simulink model "ims_Build5pt1g_tj"  (R2020b)
settings: Solver=FixedStepDiscrete  StartTime=0.0  StopTime=180  FixedStep=fem.Ts  RelTol=1e-4
InitFcn:
  | %
  | % Initialization callback function
  | %
  | 
  | try
  |    fprintf('\n New GMT IMS version!\n');
  | 
  |    % Get Simulink model directory
  |    [filepath,name,ext] = fileparts(which(bdroot));
  | 
  |    if ~strcmp(filepath,pwd)
  |       fprintf('\n Changing current directory to \n %s \n',filepath);
  |       cd(filepath);
  |    end
  | 
  |    %
  |    if(~exist('IMLoads','var'))
  |        warning('Simulation model assumes wind load is loaded...');
  |    end
  | catch
  |    warning('Running the InitFcn from puSimulate script');
  | end
values from neighbouring files (symbols this model uses):
  az = zeros(N,1)    [eval_trajectories.m]
  az_ff_en = 1    [load_IMS_5pt1g_tj.m]    (also in load_IMS_5pt1h_tj.m = 0)
  el = az    [eval_trajectories.m]
  el_ff_en = 1    [load_IMS_5pt1g_tj.m]    (also in load_IMS_5pt1h_tj.m = 0)
  fem =     [controls_5pt1g1K_z00_llTT_oad.mat]    (also in controls_5pt1g1K_z30_llTT_oad.mat)
  FEM_Ts = 1/1e3    (= 0.001)    [load_IMS_5pt1g_tj.m]    (also in load_IMS_5pt1h_tj.m)
  gir = az    [eval_trajectories.m]
  gir_ff_en = 1    [load_IMS_5pt1g_tj.m]    (also in load_IMS_5pt1h_tj.m = 0)
  H_tj = tf(1,[2*pi*0.1, 1])    [eval_trajectories.m]    (also in load_IMS_5pt1g_tj.m = c2d(Htjf,FEM_Ts, 'foh'); load_IMS_5pt1h_tj.m = c2d(Htjf,FEM_Ts, 'foh'))
  Hkin_fsm = Phi(fsm_out,1:3) * Phi_mnt_pinv    [compute_Hkin.m]
  Hkin_hp = Phi(hp_out,1:3) * Phi_mnt_pinv    [compute_Hkin.m]
  Hkin_m12 = [Phi(m1_out,1:3); Phi(m2_out,1:3)] * Phi_mnt_pinv    [compute_Hkin.m]    (also in eval_tjs.m = [Phi(m1_out,1:3); Phi(m2_out,1:3)] * pinv(Phi_mnt_enc))
  Hkin_m2p = Phi(m2p_out,1:3) * Phi_mnt_pinv    [compute_Hkin.m]
  Hkin_pmtnodes = Phi(pmt_out,1:3) * Phi_mnt_pinv    [compute_Hkin.m]    (also in eval_tjs.m = Phi(pmt_out,1:3) * pinv(Phi_mnt_enc))
  m1olf_en = 0    [load_IMS_5pt1g_tj.m]    (also in load_IMS_5pt1h_tj.m)
  m1sys =     [controls_5pt1g1K_z00_llTT_oad.mat]    (also in controls_5pt1g1K_z30_llTT_oad.mat)
  m2_pos_en = 0    [load_IMS_5pt1g_tj.m]    (also in load_IMS_5pt1h_tj.m)
  m2pos =     [controls_5pt1g1K_z00_llTT_oad.mat]    (also in controls_5pt1g1K_z30_llTT_oad.mat)
  m2pzt =     [controls_5pt1g1K_z00_llTT_oad.mat]    (also in controls_5pt1g1K_z30_llTT_oad.mat)
  m2PZT_en = 0    [load_IMS_5pt1g_tj.m]    (also in load_IMS_5pt1h_tj.m)
  mntFBc_en = 1    [load_IMS_5pt1g_tj.m]    (also in load_IMS_5pt1h_tj.m)
  mount =     [controls_5pt1g1K_z00_llTT_oad.mat]    (also in controls_5pt1g1K_z30_llTT_oad.mat; eval_tjs.m = mountY)
  om2 = (2*pi*eigenfrequencies).^2    [load_IMS_5pt1g_tj.m]    (also in load_IMS_5pt1h_tj.m)
  PG = zeros(length(om2),6)    [load_IMS_5pt1g_tj.m]    (also in load_IMS_5pt1h_tj.m)
  phiB = Phim(indDesInputs,:)'    [load_IMS_5pt1g_tj.m]    (also in load_IMS_5pt1h_tj.m)
  phiC = Phi(indDesOutputs,:)    [load_IMS_5pt1g_tj.m]    (also in load_IMS_5pt1h_tj.m)
  pmt1 = dlmread(pmt1_fname,',',[14,3,27,302])    [eval_tjs.m]    (also in eval_tjs_rtf_variants.m; load_IMS_5pt1g_tj.m; load_IMS_5pt1h_tj.m)
  pmt2 = dlmread(pmt2_fname,',',[14,3,10,302])    [eval_tjs.m]    (also in eval_tjs_rtf_variants.m; load_IMS_5pt1g_tj.m; load_IMS_5pt1h_tj.m)
  Psi_ss = gainMatrix(indDesOutputs,indDesInputs) - K_ss    [load_IMS_5pt1g_tj.m]    (also in load_IMS_5pt1h_tj.m)
  Psi_ssTs = 1/1000    (= 0.001)    [load_IMS_5pt1g_tj.m]    (also in load_IMS_5pt1h_tj.m)
  twice_zom = adjDamp*twice_zom    [load_IMS_5pt1g_tj.m]    (also in load_IMS_5pt1h_tj.m)
undefined symbols (not defined in the file or in its folder): DiscIntNeverNeededParam, magnitude
libraries: ims_block_library x20, simulink x1
(part 1 of 2)
settings Model: SimulationMode=accelerator  Creator=RRomano  LastModifiedBy=rromano
settings SolverCC: MaxConsecutiveMinStep=10  ZeroCrossAlgorithm=Adaptive
settings DataIOCC: SaveOutput=off  SignalLogging=off  DSMLogging=off  SaveTime=off  ReturnWorkspaceOutputs=off
settings OptimizationCC: DefaultParameterBehavior=Inlined  StrengthReduction=on  PassReuseOutputArgsAs=Individual arguments  EfficientMapNaN2IntZero=off  SimCompilerOptimization=on  AccelVerboseBuild=on  OptimizeBlockOrder=speed  OptimizationPriority=Speed  OptimizationCustomize=off  MultiThreadedLoops=on  EfficientTunableParamExpr=on
settings DebuggingCC: SignalInfNanChecking=warning  InheritedTsInSrcMsg=none  ParameterTunabilityLossMsg=error  SFUnexpectedBacktrackingDiag=warning  SFNoUnconditionalDefaultTransitionDiag=warning  SFExecutionAtInitializationDiag=none  ArithmeticOperatorsInVariantConditions=warning
settings HardwareCC: ProdBitPerLong=64  ProdHWDeviceType=Intel->x86-64 (Linux 64)  TargetBitPerLong=64  TargetBitPerPointer=64  TargetBitPerSizeT=64  TargetBitPerPtrDiffT=64  TargetLongLongMode=on  TargetIntDivRoundTo=Zero  TargetEndianess=LittleEndian  TargetWordSize=64  TargetHWDeviceType=MATLAB Host  ProdEqTarget=off
settings SFSimCC: SimUseLocalCustomCode=off  MATLABDynamicMemAlloc=off  CustomCodeUndefinedFunction=UseInterfaceOnly
settings RTWCC: Description=Embedded Coder  SystemTargetFile=ert.tlc  GenCodeOnly=on  TemplateMakefile=ert_default_tmf  GenerateReport=on  BuildConfiguration=Faster Runs  IncludeHyperlinkInReport=on  GenerateTraceInfo=on  GenerateTraceReport=on  GenerateTraceReportSl=on  GenerateTraceReportSf=on  GenerateTraceReportEml=on
settings CodeAppCC: ForceParamTrailComments=on  IgnoreCustomStorageClasses=off  MaxIdLength=128  OperatorAnnotations=on  SimulinkDataObjDesc=on  SFDataObjDesc=on  InsertBlockDesc=on  MATLABSourceComments=on
settings ERTTargetCC: GenerateSampleERTMain=on  InlinedParameterPlacement=NonHierarchical  ERTCustomFileTemplate=example_file_process.tlc
settings ConfigComp: CovMetricSettings=dw  CovSaveCumulativeToWorkspaceVar=on  CovSaveSingleToWorkspaceVar=on  CovExternalEMLEnable=off

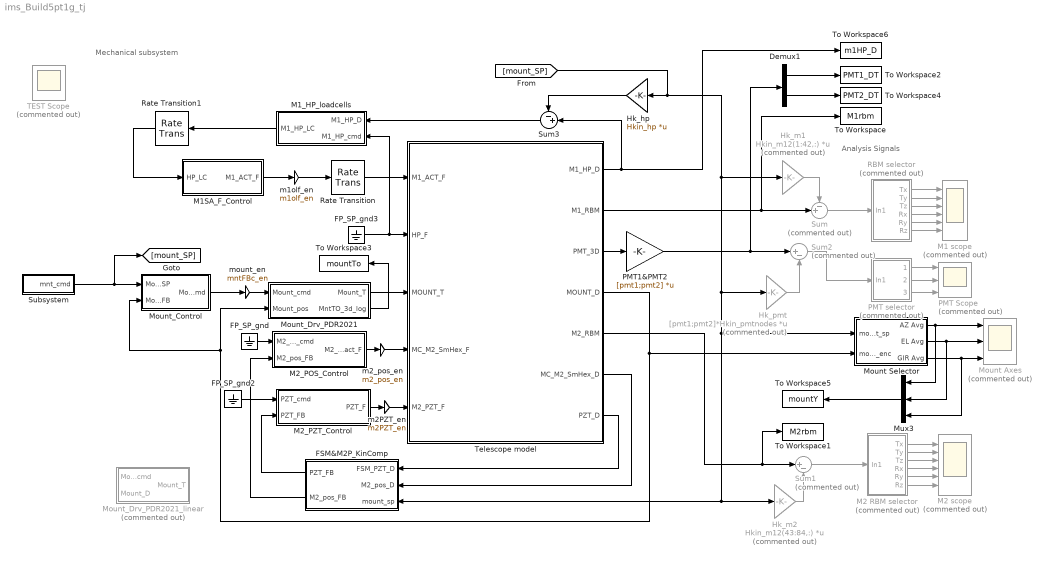
== system ims_Build5pt1g_tj ==
  note: Analysis Signals
  note: Mechanical subsystem
  Demux1 : Demux  Outputs=[14,7]
  FP_SP_gnd : Ground
  FP_SP_gnd2 : Ground
  FP_SP_gnd3 : Ground
  FSM&M2P_KinComp : Subsystem
  Hk_hp : Gain  Gain=Hkin_hp  Multiplication=Matrix(K*u)
  Hk_m1 : Gain  Commented=on  Gain=Hkin_m12(1:42,:)  Multiplication=Matrix(K*u)
  Hk_m2 : Gain  Commented=on  Gain=Hkin_m12(43:84,:)  Multiplication=Matrix(K*u)
  Hk_pmt : Gain  Commented=on  Gain=[pmt1;pmt2]*Hkin_pmtnodes  Multiplication=Matrix(K*u)
  M1 scope : Scope  Commented=on  NumInputPorts=6
  M1SA_F_Control : Subsystem
  M1_HP_loadcells : Subsystem
  M2 RBM selector : Subsystem  Commented=on
  M2 scope : Scope  Commented=on  NumInputPorts=6
  M2_POS_Control : Subsystem
  M2_PZT_Control : Subsystem
  Mount Axes : Scope  Commented=on  NumInputPorts=3
  Mount Selector : Subsystem
  Mount_Control : Subsystem
  Mount_Drv_PDR2021 : Subsystem
  Mount_Drv_PDR2021_linear : Subsystem  Commented=on
  Mux3 : Mux  Inputs=3
  PMT Scope : Scope  Commented=on  NumInputPorts=3
  PMT selector : Subsystem  Commented=on
  PMT1&PMT2 : Gain  Gain=[pmt1;pmt2]  Multiplication=Matrix(K*u)
  RBM selector : Subsystem  Commented=on
  Rate Transition : RateTransition  Deterministic=off  OutPortSampleTime=fem.Ts
  Rate Transition1 : RateTransition  Deterministic=off  OutPortSampleTime=m1sys{1}.ofl.SSdtC{1}.Ts
  Subsystem : Subsystem
  Sum : Sum  Commented=on  Inputs=-+|
  Sum1 : Sum  Commented=on  Inputs=|+-
  Sum2 : Sum  Commented=on  Inputs=|+-
  Sum3 : Sum  Inputs=-+|
  TEST Scope : Scope  Commented=on
  Telescope model : Subsystem
  To Workspace : ToWorkspace  VariableName=M1rbm  SampleTime=-1
  To Workspace1 : ToWorkspace  VariableName=M2rbm  SampleTime=-1
  To Workspace2 : ToWorkspace  VariableName=PMT1_DT  SampleTime=-1
  To Workspace3 : ToWorkspace  VariableName=mountTo  SampleTime=-1
      settings: Save2DSignal=2-D array (concatenate along first dimension)
  To Workspace4 : ToWorkspace  VariableName=PMT2_DT  SampleTime=-1
  To Workspace5 : ToWorkspace  VariableName=mountY  SaveFormat=Structure With Time  SampleTime=-1
  To Workspace6 : ToWorkspace  VariableName=m1HP_D  SampleTime=-1
  m1olf_en : Gain  Gain=m1olf_en
  m2PZT_en : Gain  Gain=m2PZT_en
  m2_pos_en : Gain  Gain=m2_pos_en
  mount_en : Gain  Gain=mntFBc_en
  wires:
  M1SA_F_Control/1(M1_ACT_F) -> m1olf_en/1
  Mount Selector/1(AZ Avg) -> Mux3/1, Mount Axes/1
  Mount Selector/2(EL Avg) -> Mux3/2, Mount Axes/2
  Mount Selector/3(GIR Avg) -> Mount Axes/3, Mux3/3
  M1_HP_loadcells/1(M1_HP_LC) -> Rate Transition1/1
  Mount_Control/1(Mount_cmd) -> mount_en/1
  RBM selector/1(Tx) -> M1 scope/1
  RBM selector/3(Tz) -> M1 scope/3
  RBM selector/4(Rx) -> M1 scope/4
  RBM selector/5(Ry) -> M1 scope/5
  RBM selector/6(Rz) -> M1 scope/6
  M2 RBM selector/1(Tx) -> M2 scope/1
  M2 RBM selector/2(Ty) -> M2 scope/2
  M2 RBM selector/3(Tz) -> M2 scope/3
  M2 RBM selector/4(Rx) -> M2 scope/4
  M2 RBM selector/5(Ry) -> M2 scope/5
  M2 RBM selector/6(Rz) -> M2 scope/6
  Telescope model/4(MOUNT_D) -> Mount Selector/2(mount_enc), Mount_Control/2(Mount_FB), Mount_Drv_PDR2021/2(Mount_pos)
  M2_PZT_Control/1(PZT_F) -> m2PZT_en/1
  M2_POS_Control/1(M2_pos_act_F) -> m2_pos_en/1
  Rate Transition/1 -> Telescope model/1(M1_ACT_F)
  FP_SP_gnd2/1 -> M2_PZT_Control/1(PZT_cmd)
  Rate Transition1/1 -> M1SA_F_Control/1(HP_LC)
  FP_SP_gnd/1 -> M2_POS_Control/1(M2_pos_cmd)
  m2_pos_en/1 -> Telescope model/4(MC_M2_SmHex_F)
  m2PZT_en/1 -> Telescope model/5(M2_PZT_F)
  m1olf_en/1 -> Rate Transition/1
  mount_en/1 -> Mount_Drv_PDR2021/1(Mount_cmd)
  FP_SP_gnd3/1 -> M1_HP_loadcells/2(M1_HP_cmd), Telescope model/2(HP_F)
  Telescope model/3(PMT_3D) -> PMT1&PMT2/1
  RBM selector/2(Ty) -> M1 scope/2
  Telescope model/2(M1_RBM) -> Sum/2, To Workspace/1
  Sum/1 -> RBM selector/1(In1)
  Telescope model/5(M2_RBM) -> To Workspace1/1, Sum1/1
  Sum1/1 -> M2 RBM selector/1(In1)
  Hk_m1/1 -> Sum/1
  Demux1/1 -> To Workspace2/1
  Demux1/2 -> To Workspace4/1
  PMT1&PMT2/1 -> Sum2/1, Demux1/1
  Sum2/1 -> PMT selector/1(In1)
  PMT selector/1(TT_Rx) -> PMT Scope/1
  PMT selector/2(TT_Ry) -> PMT Scope/2
  PMT selector/3(Piston) -> PMT Scope/3
  Mux3/1 -> To Workspace5/1
  Mount_Drv_PDR2021/1(Mount_T) -> Telescope model/3(MOUNT_T)
  Mount_Drv_PDR2021/2(MntTO_3d_log) -> To Workspace3/1
  Subsystem/1(mnt_cmd) -> [mount_SP], Mount_Control/1(Mount_SP)
  Hk_pmt/1 -> Sum2/2
  Hk_m2/1 -> Sum1/2
  Telescope model/1(M1_HP_D) -> Sum3/2, To Workspace6/1
  Sum3/1 -> M1_HP_loadcells/1(M1_HP_D)
  Hk_hp/1 -> Sum3/1
  Telescope model/7(PZT_D) -> FSM&M2P_KinComp/1(FSM_PZT_D)
  Telescope model/6(MC_M2_SmHex_D) -> FSM&M2P_KinComp/2(M2_pos_D)
  [mount_SP] -> FSM&M2P_KinComp/3(mount_sp), Hk_m2/1, Mount Selector/1(mount_sp), Hk_pmt/1, Hk_m1/1, Hk_hp/1
  FSM&M2P_KinComp/1(PZT_FB) -> M2_PZT_Control/2(PZT_FB)
  FSM&M2P_KinComp/2(M2_pos_FB) -> M2_POS_Control/2(M2_pos_FB)

== system ims_Build5pt1g_tj/FSM&M2P_KinComp ==
  FSM_PZT_D : Inport
  M2_pos_D : Inport  Port=2
  mount_sp : Inport  Port=3
  Hk_fsm : Gain  Gain=Hkin_fsm  Multiplication=Matrix(K*u)
  Hk_m2p : Gain  Gain=Hkin_m2p  Multiplication=Matrix(K*u)
  Sum4 : Sum  Inputs=|+-
  Sum5 : Sum  Inputs=|+-
  PZT_FB : Outport
  M2_pos_FB : Outport  Port=2
  wires:
  mount_sp/1 -> Hk_fsm/1, Hk_m2p/1
  FSM_PZT_D/1 -> Sum4/1
  M2_pos_D/1 -> Sum5/1
  Sum5/1 -> M2_pos_FB/1
  Sum4/1 -> PZT_FB/1
  Hk_m2p/1 -> Sum5/2
  Hk_fsm/1 -> Sum4/2

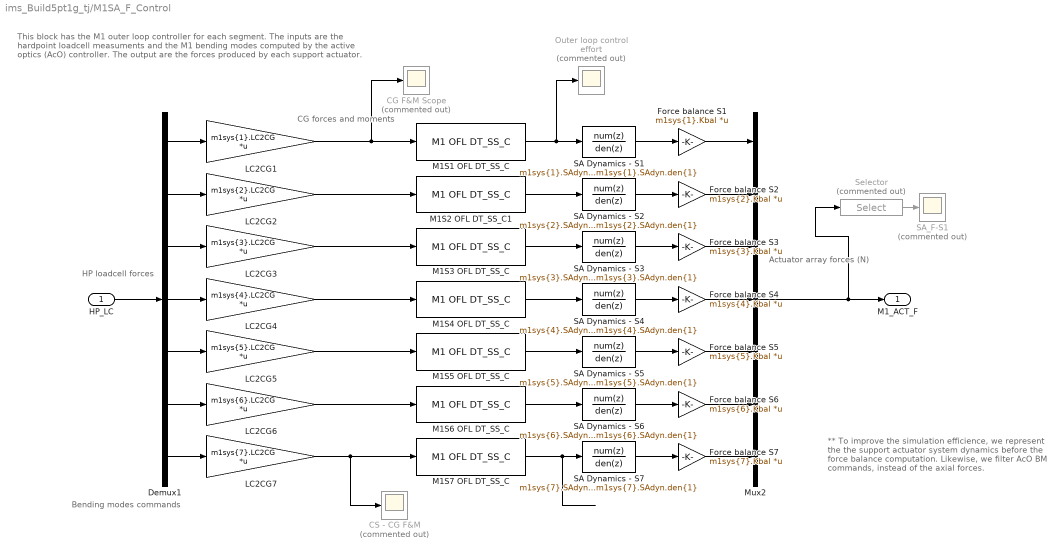
== system ims_Build5pt1g_tj/M1SA_F_Control ==
  note: HP loadcell forces
  note: This block has the M1 outer loop controller for each segment. The inputs are the hardpoint loadcell measuments and the M1 bending modes computed by the active optics (AcO) controller. The output are the forces produced by each support actuator.
  note: Actuator array
      | forces (N)
  note: CG forces
      | and moments
  note: Bending modes
      | commands
  note: ** To improve the simulation efficience, we represent the the support actuator system dynamics before the force balance computation. Likewise, we filter AcO BM commands, instead of the axial forces.
  HP_LC : Inport
  CG F&M Scope : Scope  Commented=on
  CS - CG F&M : Scope  Commented=on
  Demux1 : Demux  Outputs=6*ones(7,1)
  Force balance S1 : Gain  Gain=m1sys{1}.Kbal  Multiplication=Matrix(K*u)
  Force balance S2 : Gain  Gain=m1sys{2}.Kbal  Multiplication=Matrix(K*u)
  Force balance S3 : Gain  Gain=m1sys{3}.Kbal  Multiplication=Matrix(K*u)
  Force balance S4 : Gain  Gain=m1sys{4}.Kbal  Multiplication=Matrix(K*u)
  Force balance S5 : Gain  Gain=m1sys{5}.Kbal  Multiplication=Matrix(K*u)
  Force balance S6 : Gain  Gain=m1sys{6}.Kbal  Multiplication=Matrix(K*u)
  Force balance S7 : Gain  Gain=m1sys{7}.Kbal  Multiplication=Matrix(K*u)
  LC2CG1 : Gain  Gain=m1sys{1}.LC2CG  Multiplication=Matrix(K*u)
  LC2CG2 : Gain  Gain=m1sys{2}.LC2CG  Multiplication=Matrix(K*u)
  LC2CG3 : Gain  Gain=m1sys{3}.LC2CG  Multiplication=Matrix(K*u)
  LC2CG4 : Gain  Gain=m1sys{4}.LC2CG  Multiplication=Matrix(K*u)
  LC2CG5 : Gain  Gain=m1sys{5}.LC2CG  Multiplication=Matrix(K*u)
  LC2CG6 : Gain  Gain=m1sys{6}.LC2CG  Multiplication=Matrix(K*u)
  LC2CG7 : Gain  Gain=m1sys{7}.LC2CG  Multiplication=Matrix(K*u)
  M1S1 OFL DT_SS_C : ims_block_library/M1 OFL DT_SS_C  dt_SS_struct=m1sys{1}.ofl.SSdtC
  M1S2 OFL DT_SS_C1 : ims_block_library/M1 OFL DT_SS_C  dt_SS_struct=m1sys{2}.ofl.SSdtC
  M1S3 OFL DT_SS_C : ims_block_library/M1 OFL DT_SS_C  dt_SS_struct=m1sys{3}.ofl.SSdtC
  M1S4 OFL DT_SS_C : ims_block_library/M1 OFL DT_SS_C  dt_SS_struct=m1sys{4}.ofl.SSdtC
  M1S5 OFL DT_SS_C : ims_block_library/M1 OFL DT_SS_C  dt_SS_struct=m1sys{5}.ofl.SSdtC
  M1S6 OFL DT_SS_C : ims_block_library/M1 OFL DT_SS_C  dt_SS_struct=m1sys{6}.ofl.SSdtC
  M1S7 OFL DT_SS_C : ims_block_library/M1 OFL DT_SS_C  dt_SS_struct=m1sys{7}.ofl.SSdtC
  Mux2 : Mux  Inputs=7
  Outer loop control effort : Scope  Commented=on
  SA Dynamics - S1 : DiscreteTransferFcn  Numerator=m1sys{1}.SAdyn.num{1}  Denominator=m1sys{1}.SAdyn.den{1}  SampleTime=m1sys{1}.ofl.Ts  a0EqualsOne=on
  SA Dynamics - S2 : DiscreteTransferFcn  Numerator=m1sys{2}.SAdyn.num{1}  Denominator=m1sys{2}.SAdyn.den{1}  SampleTime=m1sys{1}.ofl.SSdtC{1}.Ts  a0EqualsOne=on
  SA Dynamics - S3 : DiscreteTransferFcn  Numerator=m1sys{3}.SAdyn.num{1}  Denominator=m1sys{3}.SAdyn.den{1}  SampleTime=m1sys{1}.ofl.SSdtC{1}.Ts  a0EqualsOne=on
  SA Dynamics - S4 : DiscreteTransferFcn  Numerator=m1sys{4}.SAdyn.num{1}  Denominator=m1sys{4}.SAdyn.den{1}  SampleTime=m1sys{1}.ofl.SSdtC{1}.Ts  a0EqualsOne=on
  SA Dynamics - S5 : DiscreteTransferFcn  Numerator=m1sys{5}.SAdyn.num{1}  Denominator=m1sys{5}.SAdyn.den{1}  SampleTime=m1sys{1}.ofl.SSdtC{1}.Ts  a0EqualsOne=on
  SA Dynamics - S6 : DiscreteTransferFcn  Numerator=m1sys{6}.SAdyn.num{1}  Denominator=m1sys{6}.SAdyn.den{1}  SampleTime=m1sys{1}.ofl.SSdtC{1}.Ts  a0EqualsOne=on
  SA Dynamics - S7 : DiscreteTransferFcn  Numerator=m1sys{7}.SAdyn.num{1}  Denominator=m1sys{7}.SAdyn.den{1}  SampleTime=m1sys{1}.ofl.SSdtC{1}.Ts  a0EqualsOne=on
  SA_F-S1 : Scope  Commented=on
  Selector : Selector  Commented=on  InputPortWidth=2316  IndexOptions=Index vector (dialog)  Indices=[1:335]  OutputSizes=1
  M1_ACT_F : Outport  VectorParamsAs1DForOutWhenUnconnected=off
  wires:
  HP_LC/1 -> Demux1/1
  M1S1 OFL DT_SS_C/1 -> Outer loop control effort/1, SA Dynamics - S1/1
  M1S2 OFL DT_SS_C1/1 -> SA Dynamics - S2/1
  M1S3 OFL DT_SS_C/1 -> SA Dynamics - S3/1
  M1S4 OFL DT_SS_C/1 -> SA Dynamics - S4/1
  M1S5 OFL DT_SS_C/1 -> SA Dynamics - S5/1
  M1S6 OFL DT_SS_C/1 -> SA Dynamics - S6/1
  M1S7 OFL DT_SS_C/1 -> SA Dynamics - S7/1
  LC2CG7/1 -> M1S7 OFL DT_SS_C/1, CS - CG F&M/1
  LC2CG6/1 -> M1S6 OFL DT_SS_C/1
  LC2CG5/1 -> M1S5 OFL DT_SS_C/1
  LC2CG4/1 -> M1S4 OFL DT_SS_C/1
  LC2CG3/1 -> M1S3 OFL DT_SS_C/1
  LC2CG2/1 -> M1S2 OFL DT_SS_C1/1
  LC2CG1/1 -> M1S1 OFL DT_SS_C/1, CG F&M Scope/1
  Demux1/1 -> LC2CG1/1
  Demux1/2 -> LC2CG2/1
  Demux1/3 -> LC2CG3/1
  Demux1/4 -> LC2CG4/1
  Demux1/5 -> LC2CG5/1
  Demux1/6 -> LC2CG6/1
  Demux1/7 -> LC2CG7/1
  Force balance S1/1 -> Mux2/1
  Force balance S2/1 -> Mux2/2
  Force balance S3/1 -> Mux2/3
  Force balance S4/1 -> Mux2/4
  Force balance S6/1 -> Mux2/6
  Force balance S5/1 -> Mux2/5
  Force balance S7/1 -> Mux2/7
  Mux2/1 -> M1_ACT_F/1, Selector/1
  SA Dynamics - S1/1 -> Force balance S1/1
  SA Dynamics - S2/1 -> Force balance S2/1
  SA Dynamics - S3/1 -> Force balance S3/1
  SA Dynamics - S4/1 -> Force balance S4/1
  SA Dynamics - S5/1 -> Force balance S5/1
  SA Dynamics - S6/1 -> Force balance S6/1
  SA Dynamics - S7/1 -> Force balance S7/1
  Selector/1 -> SA_F-S1/1

== system ims_Build5pt1g_tj/M1_HP_loadcells ==
  note: This block converts from CG displacements and rotations,
      | and converts to Hard Point lengths.  Hard point lengths are
      | changed by applying an equal and opposite force to the hard
      | point, and then offseting output by the commanded change
      | in position.
  note: Hexapod Offset Forces
  note: LC Forces (N)
  M1_HP_D : Inport
  M1_HP_cmd : Inport  Port=2
  Demux1 : Demux  Outputs=6*ones(7,1)
  Demux2 : Demux  Outputs=6*ones(14,1);%6*ones(7,1)
  M1S1 Loadcell : Subsystem
  M1S2 Loadcell : Subsystem
  M1S3 Loadcell : Subsystem
  M1S4 Loadcell : Subsystem
  M1S5 Loadcell : Subsystem
  M1S6 Loadcell : Subsystem
  M1S7 Control : Subsystem
  Mux2 : Mux  Inputs=7
  Scope : Scope  NumInputPorts=2
  M1_HP_LC : Outport  VectorParamsAs1DForOutWhenUnconnected=off
  wires:
  Demux2/9 -> M1S5 Loadcell/2(HP_D_cell)
  Demux2/3 -> M1S2 Loadcell/2(HP_D_cell)
  Demux2/5 -> M1S3 Loadcell/2(HP_D_cell)
  Demux2/13 -> M1S7 Control/2(HP_D_cell)
  Demux2/11 -> M1S6 Loadcell/2(HP_D_cell)
  Demux2/4 -> M1S2 Loadcell/3(HP_D_face)
  Demux2/6 -> M1S3 Loadcell/3(HP_D_face)
  Demux2/10 -> M1S5 Loadcell/3(HP_D_face)
  Demux2/12 -> M1S6 Loadcell/3(HP_D_face)
  Demux2/14 -> M1S7 Control/3(HP_D_face)
  M1_HP_D/1 -> Demux2/1
  M1S1 Loadcell/1(HP_F_meas) -> Mux2/1
  M1S2 Loadcell/1(HP_F_meas) -> Mux2/2
  M1S3 Loadcell/1(HP_F_meas) -> Mux2/3
  M1S5 Loadcell/1(HP_F_meas) -> Mux2/5
  M1S6 Loadcell/1(HP_F_meas) -> Mux2/6
  M1S7 Control/1(HP_F_meas) -> Mux2/7
  Demux2/2 -> M1S1 Loadcell/3(HP_D_face)
  Demux2/1 -> M1S1 Loadcell/2(HP_D_cell)
  M1S4 Loadcell/1(HP_F_meas) -> Mux2/4
  Demux2/7 -> M1S4 Loadcell/2(HP_D_cell)
  Demux2/8 -> M1S4 Loadcell/3(HP_D_face)
  M1_HP_cmd/1 -> Demux1/1
  Demux1/1 -> Scope/1, M1S1 Loadcell/1(HP_F_cmd)
  Demux1/2 -> Scope/2, M1S2 Loadcell/1(HP_F_cmd)
  Demux1/3 -> M1S3 Loadcell/1(HP_F_cmd)
  Demux1/4 -> M1S4 Loadcell/1(HP_F_cmd)
  Demux1/5 -> M1S5 Loadcell/1(HP_F_cmd)
  Demux1/6 -> M1S6 Loadcell/1(HP_F_cmd)
  Demux1/7 -> M1S7 Control/1(HP_F_cmd)
  Mux2/1 -> M1_HP_LC/1

== system ims_Build5pt1g_tj/M2 RBM selector ==
  note: Local motion of M1 segments (in m and rad)
  In1 : Inport
  Selector : Selector  InputPortWidth=42  IndexOptions=Index vector (dialog)  Indices=[1:6:42]  OutputSizes=1
  Selector1 : Selector  InputPortWidth=42  IndexOptions=Index vector (dialog)  Indices=[2:6:42]  OutputSizes=1
  Selector2 : Selector  InputPortWidth=42  IndexOptions=Index vector (dialog)  Indices=[3:6:42]  OutputSizes=1
  Selector3 : Selector  InputPortWidth=42  IndexOptions=Index vector (dialog)  Indices=[4:6:42]  OutputSizes=1
  Selector4 : Selector  InputPortWidth=42  IndexOptions=Index vector (dialog)  Indices=[5:6:42]  OutputSizes=1
  Selector5 : Selector  InputPortWidth=42  IndexOptions=Index vector (dialog)  Indices=[6:6:42]  OutputSizes=1
  Tx : Outport  VectorParamsAs1DForOutWhenUnconnected=off
  Ty : Outport  Port=2  VectorParamsAs1DForOutWhenUnconnected=off
  Tz : Outport  Port=3  VectorParamsAs1DForOutWhenUnconnected=off
  Rx : Outport  Port=4  VectorParamsAs1DForOutWhenUnconnected=off
  Ry : Outport  Port=5  VectorParamsAs1DForOutWhenUnconnected=off
  Rz : Outport  Port=6  VectorParamsAs1DForOutWhenUnconnected=off
  wires:
  In1/1 -> Selector3/1, Selector4/1, Selector5/1, Selector/1, Selector1/1, Selector2/1
  Selector/1 -> Tx/1
  Selector4/1 -> Ry/1
  Selector1/1 -> Ty/1
  Selector3/1 -> Rx/1
  Selector5/1 -> Rz/1
  Selector2/1 -> Tz/1

== system ims_Build5pt1g_tj/M2_POS_Control ==
  M2_pos_cmd : Inport
  M2_pos_FB : Inport  Port=2
  Add : Sum  Inputs=+-
  FB controller : DiscreteTransferFcn  Numerator=m2pos.fbCdt.num{1}  Denominator=m2pos.fbCdt.den{1}  SampleTime=m2pos.fbCdt.Ts
  Sel MC side : Selector  InputPortWidth=84  IndexOptions=Index vector (dialog)  Indices=[1:2:84]  OutputSizes=1
  Sel mirror side : Selector  InputPortWidth=84  IndexOptions=Index vector (dialog)  Indices=[2:2:84]  OutputSizes=1
  Sum1 : Sum  Inputs=|+-
  kron(eye(42),[1;-1]) : Gain  Gain=kron(eye(42),[1;-1])  Multiplication=Matrix(K*u) (u vector)
  M2_pos_act_F : Outport  VectorParamsAs1DForOutWhenUnconnected=off
  wires:
  FB controller/1 -> kron(eye(42),[1;-1])/1
  M2_pos_cmd/1 -> Sum1/1
  Sum1/1 -> FB controller/1
  kron(eye(42),[1;-1])/1 -> M2_pos_act_F/1
  Add/1 -> Sum1/2
  Sel MC side/1 -> Add/1
  Sel mirror side/1 -> Add/2
  M2_pos_FB/1 -> Sel mirror side/1, Sel MC side/1

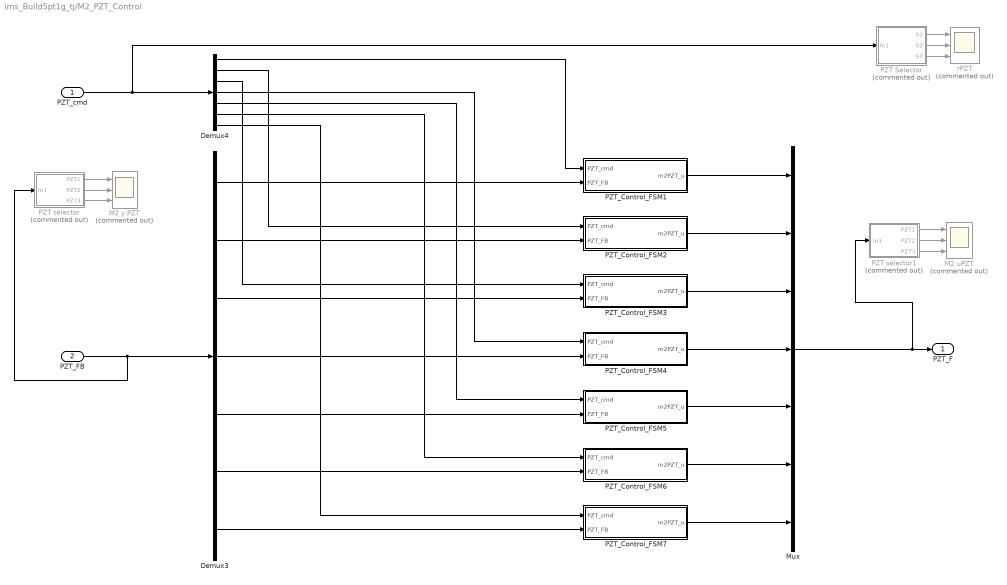
== system ims_Build5pt1g_tj/M2_PZT_Control ==
  PZT_cmd : Inport
  PZT_FB : Inport  Port=2
  Demux3 : Demux  Outputs=6*ones(7,1)
  Demux4 : Demux  Outputs=3*ones(7,1)
  M2 uPZT : Scope  Commented=on  NumInputPorts=3
  M2 y PZT : Scope  Commented=on  NumInputPorts=3
  Mux : Mux  Inputs=6*ones(1,7)
  PZT Selector : Subsystem  Commented=on
  PZT selector : Subsystem  Commented=on
  PZT selector1 : Subsystem  Commented=on
  PZT_Control_FSM1 : Subsystem
  PZT_Control_FSM2 : Subsystem
  PZT_Control_FSM3 : Subsystem
  PZT_Control_FSM4 : Subsystem
  PZT_Control_FSM5 : Subsystem
  PZT_Control_FSM6 : Subsystem
  PZT_Control_FSM7 : Subsystem
  rPZT : Scope  Commented=on  NumInputPorts=3
  PZT_F : Outport  VectorParamsAs1DForOutWhenUnconnected=off
  wires:
  Demux3/2 -> PZT_Control_FSM2/2(PZT_FB)
  Demux3/3 -> PZT_Control_FSM3/2(PZT_FB)
  Demux3/4 -> PZT_Control_FSM4/2(PZT_FB)
  Demux3/5 -> PZT_Control_FSM5/2(PZT_FB)
  Demux3/6 -> PZT_Control_FSM6/2(PZT_FB)
  Demux3/7 -> PZT_Control_FSM7/2(PZT_FB)
  PZT_FB/1 -> PZT selector/1(In1), Demux3/1
  Demux3/1 -> PZT_Control_FSM1/2(PZT_FB)
  Demux4/2 -> PZT_Control_FSM2/1(PZT_cmd)
  Demux4/3 -> PZT_Control_FSM3/1(PZT_cmd)
  Demux4/6 -> PZT_Control_FSM6/1(PZT_cmd)
  Demux4/5 -> PZT_Control_FSM5/1(PZT_cmd)
  Demux4/4 -> PZT_Control_FSM4/1(PZT_cmd)
  Demux4/7 -> PZT_Control_FSM7/1(PZT_cmd)
  Mux/1 -> PZT selector1/1(In1), PZT_F/1
  Demux4/1 -> PZT_Control_FSM1/1(PZT_cmd)
  PZT_cmd/1 -> Demux4/1, PZT Selector/1(In1)
  PZT Selector/1(S1) -> rPZT/1
  PZT Selector/2(S2) -> rPZT/2
  PZT Selector/3(S7) -> rPZT/3
  PZT selector/1(PZT1) -> M2 y PZT/1
  PZT_Control_FSM7/1(m2PZT_u) -> Mux/7
  PZT selector/2(PZT2) -> M2 y PZT/2
  PZT selector/3(PZT3) -> M2 y PZT/3
  PZT selector1/1(PZT1) -> M2 uPZT/1
  PZT selector1/2(PZT2) -> M2 uPZT/2
  PZT selector1/3(PZT3) -> M2 uPZT/3
  PZT_Control_FSM3/1(m2PZT_u) -> Mux/3
  PZT_Control_FSM1/1(m2PZT_u) -> Mux/1
  PZT_Control_FSM2/1(m2PZT_u) -> Mux/2
  PZT_Control_FSM4/1(m2PZT_u) -> Mux/4
  PZT_Control_FSM5/1(m2PZT_u) -> Mux/5
  PZT_Control_FSM6/1(m2PZT_u) -> Mux/6

== system ims_Build5pt1g_tj/Mount Selector ==
  note: Motion in rad
  mount_sp : Inport
  mount_enc : Inport  Port=2
  AzAverage : Gain  Gain=[ones(1,4)]/4  Multiplication=Matrix(K*u)
  Demux1 : Demux  Outputs=[1,1,1]
  Demux3 : Demux  Outputs=[4,6,4]
  ElAverage : Gain  Gain=[ones(1,6)]/6  Multiplication=Matrix(K*u)
  GIRAaverage : Gain  Gain=[ones(1,4)]/4  Multiplication=Matrix(K*u)
  Mux : Mux  Inputs=2
  Mux1 : Mux  Inputs=2
  Mux2 : Mux  Inputs=2
  AZ Avg : Outport  VectorParamsAs1DForOutWhenUnconnected=off
  EL Avg : Outport  Port=2  VectorParamsAs1DForOutWhenUnconnected=off
  GIR Avg : Outport  Port=3  VectorParamsAs1DForOutWhenUnconnected=off
  wires:
  Demux3/2 -> ElAverage/1
  Demux3/3 -> GIRAaverage/1
  Demux3/1 -> AzAverage/1
  mount_enc/1 -> Demux3/1
  Mux/1 -> AZ Avg/1
  AzAverage/1 -> Mux/2
  Mux1/1 -> EL Avg/1
  ElAverage/1 -> Mux1/2
  GIRAaverage/1 -> Mux2/2
  Mux2/1 -> GIR Avg/1
  mount_sp/1 -> Demux1/1
  Demux1/3 -> Mux2/1
  Demux1/1 -> Mux/1
  Demux1/2 -> Mux1/1

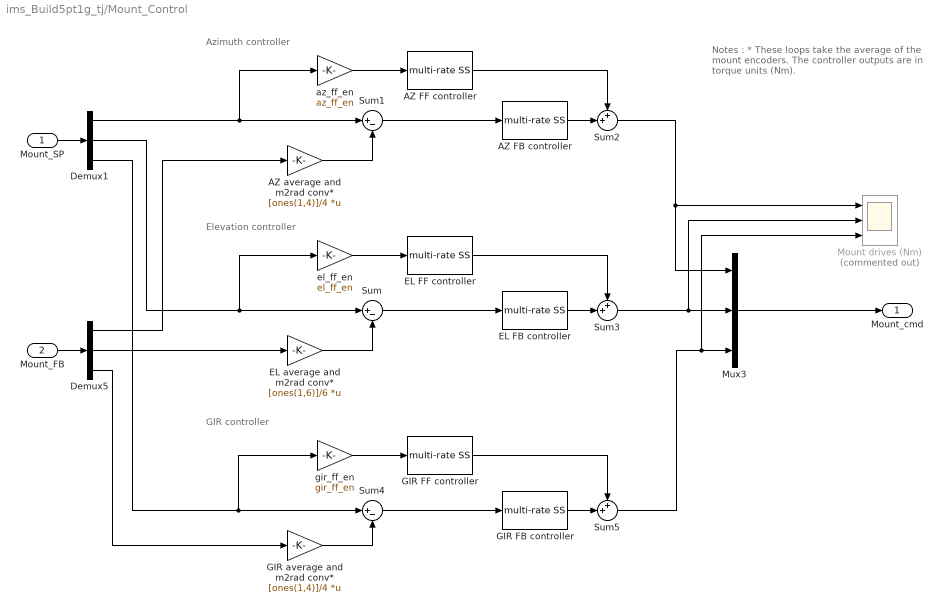
== system ims_Build5pt1g_tj/Mount_Control ==
  note: GIR controller
  note: Elevation controller
  note: Azimuth controller
  note: Notes :
      | * These loops take the average of the mount encoders. The controller outputs are in torque units (Nm).
  Mount_SP : Inport
  Mount_FB : Inport  Port=2
  AZ FB controller : ims_block_library/multi-rate SS  ss_model=mount.az.SSdtHfb
  AZ FF controller : ims_block_library/multi-rate SS  ss_model=mount.az.SSdtHff
  AZ average and m2rad conv* : Gain  Gain=[ones(1,4)]/4  Multiplication=Matrix(K*u)
  Demux1 : Demux  Outputs=[1,1,1]
  Demux5 : Demux  Outputs=[4,6,4]
  EL FB controller : ims_block_library/multi-rate SS  ss_model=mount.el.SSdtHfb
  EL FF controller : ims_block_library/multi-rate SS  ss_model=mount.el.SSdtHff
  EL average and m2rad conv* : Gain  Gain=[ones(1,6)]/6  Multiplication=Matrix(K*u)
  GIR FB controller : ims_block_library/multi-rate SS  ss_model=mount.gir.SSdtHfb
  GIR FF controller : ims_block_library/multi-rate SS  ss_model=mount.gir.SSdtHff
  GIR average and m2rad conv* : Gain  Gain=[ones(1,4)]/4  Multiplication=Matrix(K*u)
  Mount drives (Nm) : Scope  Commented=on  NumInputPorts=3
  Mux3 : Mux  Inputs=[1,1,1]
  Sum : Sum  Inputs=|+-
  Sum1 : Sum  Inputs=|+-
  Sum2 : Sum  Inputs=++|
  Sum3 : Sum  Inputs=++|
  Sum4 : Sum  Inputs=|+-
  Sum5 : Sum  Inputs=++|
  az_ff_en : Gain  Gain=az_ff_en
  el_ff_en : Gain  Gain=el_ff_en
  gir_ff_en : Gain  Gain=gir_ff_en
  Mount_cmd : Outport  VectorParamsAs1DForOutWhenUnconnected=off
  wires:
  Mount_FB/1 -> Demux5/1
  Sum1/1 -> AZ FB controller/1
  Demux1/3 -> gir_ff_en/1, Sum4/1
  AZ average and m2rad conv*/1 -> Sum1/2
  EL average and m2rad conv*/1 -> Sum/2
  Mount_SP/1 -> Demux1/1
  Demux1/1 -> az_ff_en/1, Sum1/1
  Demux1/2 -> el_ff_en/1, Sum/1
  Sum/1 -> EL FB controller/1
  Sum4/1 -> GIR FB controller/1
  Demux5/1 -> AZ average and m2rad conv*/1
  Demux5/2 -> EL average and m2rad conv*/1
  GIR average and m2rad conv*/1 -> Sum4/2
  Demux5/3 -> GIR average and m2rad conv*/1
  Mux3/1 -> Mount_cmd/1
  AZ FB controller/1 -> Sum2/2
  az_ff_en/1 -> AZ FF controller/1
  AZ FF controller/1 -> Sum2/1
  Sum2/1 -> Mount drives (Nm)/1, Mux3/1
  EL FB controller/1 -> Sum3/2
  Sum3/1 -> Mount drives (Nm)/2, Mux3/2
  EL FF controller/1 -> Sum3/1
  el_ff_en/1 -> EL FF controller/1
  gir_ff_en/1 -> GIR FF controller/1
  GIR FB controller/1 -> Sum5/2
  Sum5/1 -> Mount drives (Nm)/3, Mux3/3
  GIR FF controller/1 -> Sum5/1

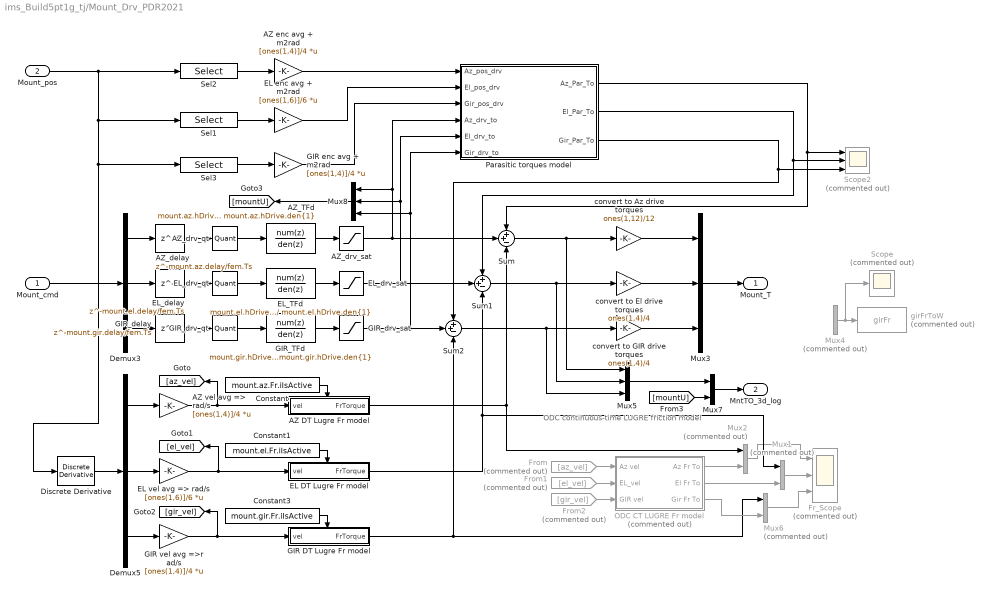
== system ims_Build5pt1g_tj/Mount_Drv_PDR2021 ==
  note: ODC continuous-time LUGRE friction model
  Mount_cmd : Inport
  Mount_pos : Inport  Port=2
  AZ DT Lugre Fr model : Subsystem  TreatAsAtomicUnit=on  mask{frParStruct=mount.az.Fr}
      mask prompts: frParStruct "Structure with the Friction model parameters"
  AZ enc avg + m2rad : Gain  Gain=[ones(1,4)]/4  Multiplication=Matrix(K*u)
  AZ vel avg => rad/s : Gain  Gain=[ones(1,4)]/4  Multiplication=Matrix(K*u)
  AZ_TFd : DiscreteTransferFcn  Numerator=mount.az.hDrive.num{1}  Denominator=mount.az.hDrive.den{1}  SampleTime=mount.el.hDrive.Ts  a0EqualsOne=on
  AZ_delay : Delay  DelayLength=mount.az.delay/fem.Ts  UseCircularBuffer=on  SampleTime=mount.az.hDrive.Ts
  AZ_drv_qt : Quantizer  QuantizationInterval=mount.az.driveQuant
  AZ_drv_sat : Saturate  UpperLimit=mount.az.Tmax  LowerLimit=-mount.az.Tmax
  Constant : Constant  Value=mount.az.Fr.iIsActive
  Constant1 : Constant  Value=mount.el.Fr.iIsActive
  Constant3 : Constant  Value=mount.gir.Fr.iIsActive
  Demux3 : Demux  Outputs=3
  Demux5 : Demux  Outputs=[4,6,4]
  Discrete Derivative : simulink/Discrete/Discrete Derivative  gainval=1  ICPrevScaledInput=0.0  OutMin=[]  OutMax=[]  OutDataType=fixdt(1, 16)  OutScaling=2^-10  DoSatur=off
  EL DT Lugre Fr model : Subsystem  TreatAsAtomicUnit=on  mask{frParStruct=mount.el.Fr}
      mask prompts: frParStruct "Structure with the Friction model parameters"
  EL enc avg + m2rad : Gain  Gain=[ones(1,6)]/6  Multiplication=Matrix(K*u)
  EL vel avg => rad/s : Gain  Gain=[ones(1,6)]/6  Multiplication=Matrix(K*u)
  EL_TFd : DiscreteTransferFcn  Numerator=mount.el.hDrive.num{1}  Denominator=mount.el.hDrive.den{1}  SampleTime=mount.el.hDrive.Ts  a0EqualsOne=on
  EL_delay : Delay  DelayLength=mount.el.delay/fem.Ts  UseCircularBuffer=on  SampleTime=mount.el.hDrive.Ts
  EL_drv_qt : Quantizer  QuantizationInterval=mount.el.driveQuant
  EL_drv_sat : Saturate  UpperLimit=mount.el.Tmax  LowerLimit=-mount.el.Tmax
  Fr_Scope : Scope  Commented=on  NumInputPorts=3
  From : From  Commented=on  GotoTag=az_vel
  From1 : From  Commented=on  GotoTag=el_vel
  From2 : From  Commented=on  GotoTag=gir_vel
  GIR DT Lugre Fr model : Subsystem  TreatAsAtomicUnit=on  mask{frParStruct=mount.gir.Fr}
      mask prompts: frParStruct "Structure with the Friction model parameters"
  GIR enc avg + m2rad : Gain  Gain=[ones(1,4)]/4  Multiplication=Matrix(K*u)
  GIR vel avg =>r ad/s : Gain  Gain=[ones(1,4)]/4  Multiplication=Matrix(K*u)
  GIR_TFd : DiscreteTransferFcn  Numerator=mount.gir.hDrive.num{1}  Denominator=mount.gir.hDrive.den{1}  SampleTime=mount.gir.hDrive.Ts  a0EqualsOne=on
  GIR_delay : Delay  DelayLength=mount.gir.delay/fem.Ts  UseCircularBuffer=on  SampleTime=mount.gir.hDrive.Ts
  GIR_drv_qt : Quantizer  QuantizationInterval=mount.gir.driveQuant
  GIR_drv_sat : Saturate  UpperLimit=mount.gir.Tmax  LowerLimit=-mount.gir.Tmax
  Mux1 : Mux  Commented=on  Inputs=2
  Mux2 : Mux  Commented=on  Inputs=2
  Mux3 : Mux  Inputs=[12,4,4]
  Mux4 : Mux  Commented=on  Inputs=3
  Mux5 : Mux  Inputs=3
  Mux6 : Mux  Commented=on  Inputs=2
  Mux7 : Mux  Inputs=2
  Mux8 : Mux  Inputs=3
  ODC CT LUGRE Fr model : Subsystem  Commented=on
  "Parasitic torques model " : Subsystem
  Scope : Scope  Commented=on
  Scope2 : Scope  Commented=on  NumInputPorts=3
  Sel1 : Selector  InputPortWidth=14  IndexOptions=Index vector (dialog)  Indices=[5:10]  OutputSizes=1
  Sel2 : Selector  InputPortWidth=14  IndexOptions=Index vector (dialog)  Indices=[1:4]  OutputSizes=1
  Sel3 : Selector  InputPortWidth=14  IndexOptions=Index vector (dialog)  Indices=[11:14]  OutputSizes=1
  Sum : Sum  Inputs=++-
  Sum1 : Sum  Inputs=++-
  Sum2 : Sum  Inputs=++-
  convert to Az drive torques : Gain  Gain=ones(1,12)/12
  convert to El drive torques : Gain  Gain=ones(1,4)/4
  convert to GIR drive torques : Gain  Gain=ones(1,4)/4
  girFrToW : ToWorkspace  Commented=on  VariableName=girFr  SaveFormat=Structure With Time  SampleTime=-1
  Mount_T : Outport  VectorParamsAs1DForOutWhenUnconnected=off
  MntTO_3d_log : Outport  Port=2  VectorParamsAs1DForOutWhenUnconnected=off
  wires:
  EL_TFd/1 -> EL_drv_sat/1
  AZ_TFd/1 -> AZ_drv_sat/1
  Mux3/1 -> Mount_T/1
  convert to Az drive torques/1 -> Mux3/1
  convert to El drive torques/1 -> Mux3/2
  convert to GIR drive torques/1 -> Mux3/3
  Demux3/2 -> EL_delay/1
  Demux3/1 -> AZ_delay/1
  AZ_delay/1 -> AZ_drv_qt/1
  EL_delay/1 -> EL_drv_qt/1
  AZ_drv_qt/1 -> AZ_TFd/1
  EL_drv_qt/1 -> EL_TFd/1
  Demux5/1 -> AZ vel avg => rad/s/1
  Demux5/2 -> EL vel avg => rad/s/1
  Demux5/3 -> GIR vel avg =>r ad/s/1
  Discrete Derivative/1 -> Demux5/1
  AZ vel avg => rad/s/1 -> [az_vel], AZ DT Lugre Fr model/1(vel)
  Constant/1 -> AZ DT Lugre Fr model/Enable
  Mux2/1 -> Fr_Scope/1
  AZ DT Lugre Fr model/1(FrTorque) -> Sum/3, Mux2/1
  EL_drv_sat/1 -> Mux8/2, "Parasitic torques model "/5(El_drv_to), Sum1/2
  EL DT Lugre Fr model/1(FrTorque) -> Sum1/3, Mux1/1
  Mux1/1 -> Fr_Scope/2
  Sel2/1 -> AZ enc avg + m2rad/1
  Sel1/1 -> EL enc avg + m2rad/1
  Mount_pos/1 -> Sel2/1, Discrete Derivative/1, Sel3/1, Sel1/1
  AZ_drv_sat/1 -> Mux8/1, "Parasitic torques model "/4(Az_drv_to), Sum/2
  Demux3/3 -> GIR_delay/1
  GIR_TFd/1 -> GIR_drv_sat/1
  GIR_delay/1 -> GIR_drv_qt/1
  GIR_drv_qt/1 -> GIR_TFd/1
  GIR_drv_sat/1 -> Mux8/3, "Parasitic torques model "/6(Gir_drv_to), Sum2/2
  Constant3/1 -> GIR DT Lugre Fr model/Enable
  Sel3/1 -> GIR enc avg + m2rad/1
  AZ enc avg + m2rad/1 -> "Parasitic torques model "/1(Az_pos_drv)
  EL enc avg + m2rad/1 -> "Parasitic torques model "/2(El_pos_drv)
  GIR enc avg + m2rad/1 -> "Parasitic torques model "/3(Gir_pos_drv)
  Sum/1 -> Mux5/1, convert to Az drive torques/1
  Sum1/1 -> Mux5/2, convert to El drive torques/1
  Sum2/1 -> Mux5/3, convert to GIR drive torques/1
  Constant1/1 -> EL DT Lugre Fr model/Enable
  GIR vel avg =>r ad/s/1 -> [gir_vel], GIR DT Lugre Fr model/1(vel)
  "Parasitic torques model "/1(Az_Par_To) -> Scope2/1, Sum/1
  "Parasitic torques model "/2(El_Par_To) -> Scope2/2, Sum1/1
  "Parasitic torques model "/3(Gir_Par_To) -> Sum2/1, Scope2/3
  GIR DT Lugre Fr model/1(FrTorque) -> Sum2/3, Mux6/1
  Mux6/1 -> Fr_Scope/3
  EL vel avg => rad/s/1 -> [el_vel], EL DT Lugre Fr model/1(vel)
  ODC CT LUGRE Fr model/1(Az Fr To) -> Mux2/2
  ODC CT LUGRE Fr model/2(El Fr To) -> Mux1/2
  Mount_cmd/1 -> Demux3/1
  From/1 -> ODC CT LUGRE Fr model/1(Az vel)
  From1/1 -> ODC CT LUGRE Fr model/2(EL_vel)
  From2/1 -> ODC CT LUGRE Fr model/3(GIR vel)
  ODC CT LUGRE Fr model/3(Gir Fr To) -> Mux6/2
  Mux4/1 -> Scope/1, girFrToW/1
  Mux5/1 -> Mux7/1
  Mux8/1 -> [mountU]
  Mux7/1 -> MntTO_3d_log/1
  [mountU] -> Mux7/2

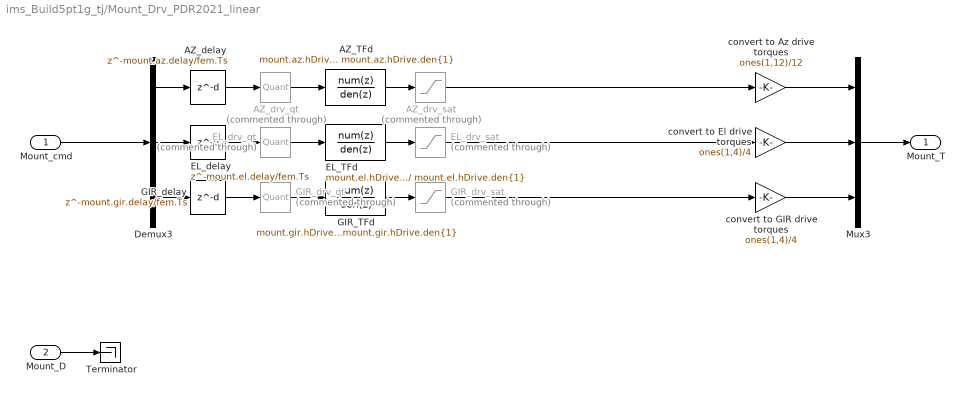
== system ims_Build5pt1g_tj/Mount_Drv_PDR2021_linear ==
  Mount_cmd : Inport
  Mount_D : Inport  Port=2
  AZ_TFd : DiscreteTransferFcn  Numerator=mount.az.hDrive.num{1}  Denominator=mount.az.hDrive.den{1}  SampleTime=mount.el.hDrive.Ts  a0EqualsOne=on
  AZ_delay : Delay  DelayLength=mount.az.delay/fem.Ts  UseCircularBuffer=on  SampleTime=mount.az.hDrive.Ts
  AZ_drv_qt : Quantizer  Commented=through  QuantizationInterval=mount.az.driveQuant
  AZ_drv_sat : Saturate  Commented=through  UpperLimit=mount.az.Tmax  LowerLimit=-mount.az.Tmax
  Demux3 : Demux  Outputs=3
  EL_TFd : DiscreteTransferFcn  Numerator=mount.el.hDrive.num{1}  Denominator=mount.el.hDrive.den{1}  SampleTime=mount.el.hDrive.Ts  a0EqualsOne=on
  EL_delay : Delay  DelayLength=mount.el.delay/fem.Ts  UseCircularBuffer=on  SampleTime=mount.el.hDrive.Ts
  EL_drv_qt : Quantizer  Commented=through  QuantizationInterval=mount.el.driveQuant
  EL_drv_sat : Saturate  Commented=through  UpperLimit=mount.el.Tmax  LowerLimit=-mount.el.Tmax
  GIR_TFd : DiscreteTransferFcn  Numerator=mount.gir.hDrive.num{1}  Denominator=mount.gir.hDrive.den{1}  SampleTime=mount.gir.hDrive.Ts  a0EqualsOne=on
  GIR_delay : Delay  DelayLength=mount.gir.delay/fem.Ts  UseCircularBuffer=on  SampleTime=mount.gir.hDrive.Ts
  GIR_drv_qt : Quantizer  Commented=through  QuantizationInterval=mount.gir.driveQuant
  GIR_drv_sat : Saturate  Commented=through  UpperLimit=mount.gir.Tmax  LowerLimit=-mount.gir.Tmax
  Mux3 : Mux  Inputs=[12,4,4]
  Terminator : Terminator
  convert to Az drive torques : Gain  Gain=ones(1,12)/12
  convert to El drive torques : Gain  Gain=ones(1,4)/4
  convert to GIR drive torques : Gain  Gain=ones(1,4)/4
  Mount_T : Outport  VectorParamsAs1DForOutWhenUnconnected=off
  wires:
  EL_TFd/1 -> EL_drv_sat/1
  AZ_TFd/1 -> AZ_drv_sat/1
  Mux3/1 -> Mount_T/1
  convert to Az drive torques/1 -> Mux3/1
  convert to El drive torques/1 -> Mux3/2
  convert to GIR drive torques/1 -> Mux3/3
  Demux3/2 -> EL_delay/1
  Demux3/1 -> AZ_delay/1
  AZ_delay/1 -> AZ_drv_qt/1
  EL_delay/1 -> EL_drv_qt/1
  AZ_drv_qt/1 -> AZ_TFd/1
  EL_drv_qt/1 -> EL_TFd/1
  Demux3/3 -> GIR_delay/1
  GIR_TFd/1 -> GIR_drv_sat/1
  GIR_delay/1 -> GIR_drv_qt/1
  GIR_drv_qt/1 -> GIR_TFd/1
  GIR_drv_sat/1 -> convert to GIR drive torques/1
  Mount_cmd/1 -> Demux3/1
  EL_drv_sat/1 -> convert to El drive torques/1
  AZ_drv_sat/1 -> convert to Az drive torques/1
  Mount_D/1 -> Terminator/1

== system ims_Build5pt1g_tj/PMT selector ==
  note: Local motion of M1 segments (in m and rad)
  In1 : Inport
  Selector : Selector  InputPortWidth=21  IndexOptions=Index vector (dialog)  Indices=[1:2:14]  OutputSizes=1
  Selector1 : Selector  InputPortWidth=21  IndexOptions=Index vector (dialog)  Indices=[2:2:14]  OutputSizes=1
  Selector2 : Selector  InputPortWidth=21  IndexOptions=Index vector (dialog)  Indices=[15:21]  OutputSizes=1
  TT_Rx : Outport  VectorParamsAs1DForOutWhenUnconnected=off
  TT_Ry : Outport  Port=2  VectorParamsAs1DForOutWhenUnconnected=off
  Piston : Outport  Port=3  VectorParamsAs1DForOutWhenUnconnected=off
  wires:
  In1/1 -> Selector/1, Selector1/1, Selector2/1
  Selector/1 -> TT_Rx/1
  Selector1/1 -> TT_Ry/1
  Selector2/1 -> Piston/1

== system ims_Build5pt1g_tj/RBM selector ==
  note: Local motion of M1 segments (in m and rad)
  In1 : Inport
  Selector : Selector  InputPortWidth=42  IndexOptions=Index vector (dialog)  Indices=[1:6:42]  OutputSizes=1
  Selector1 : Selector  InputPortWidth=42  IndexOptions=Index vector (dialog)  Indices=[2:6:42]  OutputSizes=1
  Selector2 : Selector  InputPortWidth=42  IndexOptions=Index vector (dialog)  Indices=[3:6:42]  OutputSizes=1
  Selector3 : Selector  InputPortWidth=42  IndexOptions=Index vector (dialog)  Indices=[4:6:42]  OutputSizes=1
  Selector4 : Selector  InputPortWidth=42  IndexOptions=Index vector (dialog)  Indices=[5:6:42]  OutputSizes=1
  Selector5 : Selector  InputPortWidth=42  IndexOptions=Index vector (dialog)  Indices=[6:6:42]  OutputSizes=1
  Tx : Outport  VectorParamsAs1DForOutWhenUnconnected=off
  Ty : Outport  Port=2  VectorParamsAs1DForOutWhenUnconnected=off
  Tz : Outport  Port=3  VectorParamsAs1DForOutWhenUnconnected=off
  Rx : Outport  Port=4  VectorParamsAs1DForOutWhenUnconnected=off
  Ry : Outport  Port=5  VectorParamsAs1DForOutWhenUnconnected=off
  Rz : Outport  Port=6  VectorParamsAs1DForOutWhenUnconnected=off
  wires:
  In1/1 -> Selector3/1, Selector4/1, Selector5/1, Selector/1, Selector1/1, Selector2/1
  Selector/1 -> Tx/1
  Selector4/1 -> Ry/1
  Selector1/1 -> Ty/1
  Selector3/1 -> Rx/1
  Selector5/1 -> Rz/1
  Selector2/1 -> Tz/1

== system ims_Build5pt1g_tj/Subsystem ==
  Mount_Tj : FromWorkspace  VariableName=mount_tj  SampleTime=-1  OutputAfterFinalValue=Holding final value
  TJ Filter : DiscreteTransferFcn  Numerator=H_tj.num{1}  Denominator=H_tj.den{1}  SampleTime=H_tj.Ts
  mnt_cmd : Outport
  wires:
  TJ Filter/1 -> mnt_cmd/1
  Mount_Tj/1 -> TJ Filter/1

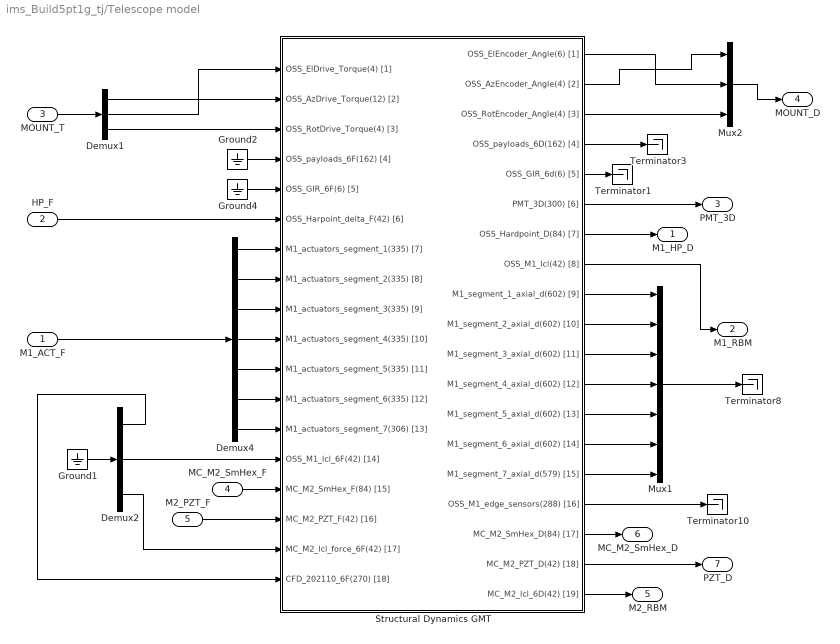
== system ims_Build5pt1g_tj/Telescope model ==
  M1_ACT_F : Inport
  HP_F : Inport  Port=2
  MOUNT_T : Inport  Port=3
  MC_M2_SmHex_F : Inport  Port=4
  M2_PZT_F : Inport  Port=5
  Demux1 : Demux  Outputs=[12,4,4]
  Demux2 : Demux  Outputs=[270,42,42]
  Demux4 : Demux  Outputs=[335,335,335,335,335,335,306]
  Ground1 : Ground
  Ground2 : Ground
  Ground4 : Ground
  Mux1 : Mux  Inputs=7
  Mux2 : Mux  Inputs=[4,6,4]
  Structural Dynamics GMT : Subsystem
  Terminator{1,3,8,10} (4 alike) : Terminator
  M1_HP_D : Outport  VectorParamsAs1DForOutWhenUnconnected=off
  M1_RBM : Outport  Port=2  VectorParamsAs1DForOutWhenUnconnected=off
  PMT_3D : Outport  Port=3  VectorParamsAs1DForOutWhenUnconnected=off
  MOUNT_D : Outport  Port=4  VectorParamsAs1DForOutWhenUnconnected=off
  M2_RBM : Outport  Port=5  VectorParamsAs1DForOutWhenUnconnected=off
  MC_M2_SmHex_D : Outport  Port=6  VectorParamsAs1DForOutWhenUnconnected=off
  PZT_D : Outport  Port=7  VectorParamsAs1DForOutWhenUnconnected=off
  wires:
  Demux4/3 -> Structural Dynamics GMT/9(M1_actuators_segment_3(335) [9])
  Demux1/3 -> Structural Dynamics GMT/3(OSS_RotDrive_Torque(4) [3])
  Structural Dynamics GMT/4(OSS_payloads_6D(162) [4]) -> Terminator3/1
  Demux4/7 -> Structural Dynamics GMT/13(M1_actuators_segment_7(306) [13])
  Demux4/1 -> Structural Dynamics GMT/7(M1_actuators_segment_1(335) [7])
  Demux4/6 -> Structural Dynamics GMT/12(M1_actuators_segment_6(335) [12])
  Structural Dynamics GMT/3(OSS_RotEncoder_Angle(4) [3]) -> Mux2/3
  M2_PZT_F/1 -> Structural Dynamics GMT/16(MC_M2_PZT_F(42) [16])
  Mux2/1 -> MOUNT_D/1
  Demux4/4 -> Structural Dynamics GMT/10(M1_actuators_segment_4(335) [10])
  Demux4/5 -> Structural Dynamics GMT/11(M1_actuators_segment_5(335) [11])
  M1_ACT_F/1 -> Demux4/1
  Structural Dynamics GMT/18(MC_M2_PZT_D(42) [18]) -> PZT_D/1
  Demux4/2 -> Structural Dynamics GMT/8(M1_actuators_segment_2(335) [8])
  Mux1/1 -> Terminator8/1
  MOUNT_T/1 -> Demux1/1
  Structural Dynamics GMT/19(MC_M2_lcl_6D(42) [19]) -> M2_RBM/1
  HP_F/1 -> Structural Dynamics GMT/6(OSS_Harpoint_delta_F(42) [6])
  Structural Dynamics GMT/7(OSS_Hardpoint_D(84) [7]) -> M1_HP_D/1
  Structural Dynamics GMT/5(OSS_GIR_6d(6) [5]) -> Terminator1/1
  Demux1/1 -> Structural Dynamics GMT/2(OSS_AzDrive_Torque(12) [2])
  Demux1/2 -> Structural Dynamics GMT/1(OSS_ElDrive_Torque(4) [1])
  Structural Dynamics GMT/1(OSS_ElEncoder_Angle(6) [1]) -> Mux2/2
  Structural Dynamics GMT/2(OSS_AzEncoder_Angle(4) [2]) -> Mux2/1
  MC_M2_SmHex_F/1 -> Structural Dynamics GMT/15(MC_M2_SmHex_F(84) [15])
  Structural Dynamics GMT/8(OSS_M1_lcl(42) [8]) -> M1_RBM/1
  Structural Dynamics GMT/16(OSS_M1_edge_sensors(288) [16]) -> Terminator10/1
  Structural Dynamics GMT/17(MC_M2_SmHex_D(84) [17]) -> MC_M2_SmHex_D/1
  Structural Dynamics GMT/9(M1_segment_1_axial_d(602) [9]) -> Mux1/1
  Structural Dynamics GMT/10(M1_segment_2_axial_d(602) [10]) -> Mux1/2
  Structural Dynamics GMT/11(M1_segment_3_axial_d(602) [11]) -> Mux1/3
  Structural Dynamics GMT/12(M1_segment_4_axial_d(602) [12]) -> Mux1/4
  Structural Dynamics GMT/13(M1_segment_5_axial_d(602) [13]) -> Mux1/5
  Structural Dynamics GMT/14(M1_segment_6_axial_d(602) [14]) -> Mux1/6
  Structural Dynamics GMT/15(M1_segment_7_axial_d(579) [15]) -> Mux1/7
  Ground2/1 -> Structural Dynamics GMT/4(OSS_payloads_6F(162) [4])
  Ground4/1 -> Structural Dynamics GMT/5(OSS_GIR_6F(6) [5])
  Demux2/3 -> Structural Dynamics GMT/17(MC_M2_lcl_force_6F(42) [17])
  Demux2/2 -> Structural Dynamics GMT/14(OSS_M1_lcl_6F(42) [14])
  Structural Dynamics GMT/6(PMT_3D(300) [6]) -> PMT_3D/1
  Ground1/1 -> Demux2/1
  Demux2/1 -> Structural Dynamics GMT/18(CFD_202110_6F(270) [18])

== system ims_Build5pt1g_tj/M1_HP_loadcells/M1S1 Loadcell ==
  note: HP Forces
  note: HP Relative
      | Displacements
  HP_F_cmd : Inport
  HP_D_cell : Inport  Port=2
  HP_D_face : Inport  Port=3
  HpK : Gain  Gain=m1sys{1}.HPstiff
  Sum1 : Sum  Inputs=-+|
  Sum9 : Sum  Inputs=-+|
  HP_F_meas : Outport  VectorParamsAs1DForOutWhenUnconnected=off
  wires:
  HP_D_cell/1 -> Sum9/1
  HP_D_face/1 -> Sum9/2
  Sum9/1 -> HpK/1
  HpK/1 -> Sum1/2
  Sum1/1 -> HP_F_meas/1
  HP_F_cmd/1 -> Sum1/1

== system ims_Build5pt1g_tj/M1_HP_loadcells/M1S2 Loadcell ==
  note: HP Relative
      | Displacements
  note: HP Forces
  HP_F_cmd : Inport
  HP_D_cell : Inport  Port=2
  HP_D_face : Inport  Port=3
  HpK : Gain  Gain=m1sys{2}.HPstiff
  Sum1 : Sum  Inputs=-+|
  Sum9 : Sum  Inputs=-+|
  HP_F_meas : Outport  VectorParamsAs1DForOutWhenUnconnected=off
  wires:
  HP_D_face/1 -> Sum9/2
  HP_D_cell/1 -> Sum9/1
  HP_F_cmd/1 -> Sum1/1
  HpK/1 -> Sum1/2
  Sum1/1 -> HP_F_meas/1
  Sum9/1 -> HpK/1

== system ims_Build5pt1g_tj/M1_HP_loadcells/M1S3 Loadcell ==
  note: HP Relative
      | Displacements
  note: HP Forces
  HP_F_cmd : Inport
  HP_D_cell : Inport  Port=2
  HP_D_face : Inport  Port=3
  HpK : Gain  Gain=m1sys{3}.HPstiff
  Sum1 : Sum  Inputs=-+|
  Sum9 : Sum  Inputs=-+|
  HP_F_meas : Outport  VectorParamsAs1DForOutWhenUnconnected=off
  wires:
  HP_D_face/1 -> Sum9/2
  HP_D_cell/1 -> Sum9/1
  HP_F_cmd/1 -> Sum1/1
  HpK/1 -> Sum1/2
  Sum1/1 -> HP_F_meas/1
  Sum9/1 -> HpK/1

== system ims_Build5pt1g_tj/M1_HP_loadcells/M1S4 Loadcell ==
  note: HP Relative
      | Displacements
  note: HP Forces
  HP_F_cmd : Inport
  HP_D_cell : Inport  Port=2
  HP_D_face : Inport  Port=3
  HpK : Gain  Gain=m1sys{4}.HPstiff
  Sum1 : Sum  Inputs=-+|
  Sum9 : Sum  Inputs=-+|
  HP_F_meas : Outport  VectorParamsAs1DForOutWhenUnconnected=off
  wires:
  HP_D_face/1 -> Sum9/2
  HP_D_cell/1 -> Sum9/1
  HP_F_cmd/1 -> Sum1/1
  HpK/1 -> Sum1/2
  Sum1/1 -> HP_F_meas/1
  Sum9/1 -> HpK/1

== system ims_Build5pt1g_tj/M1_HP_loadcells/M1S5 Loadcell ==
  note: HP Relative
      | Displacements
  note: HP Forces
  HP_F_cmd : Inport
  HP_D_cell : Inport  Port=2
  HP_D_face : Inport  Port=3
  HpK : Gain  Gain=m1sys{5}.HPstiff
  Sum1 : Sum  Inputs=-+|
  Sum9 : Sum  Inputs=-+|
  HP_F_meas : Outport  VectorParamsAs1DForOutWhenUnconnected=off
  wires:
  HP_D_face/1 -> Sum9/2
  HP_D_cell/1 -> Sum9/1
  HP_F_cmd/1 -> Sum1/1
  HpK/1 -> Sum1/2
  Sum1/1 -> HP_F_meas/1
  Sum9/1 -> HpK/1

== system ims_Build5pt1g_tj/M1_HP_loadcells/M1S6 Loadcell ==
  note: HP Relative
      | Displacements
  note: HP Forces
  HP_F_cmd : Inport
  HP_D_cell : Inport  Port=2
  HP_D_face : Inport  Port=3
  HpK : Gain  Gain=m1sys{6}.HPstiff
  Sum1 : Sum  Inputs=-+|
  Sum9 : Sum  Inputs=-+|
  HP_F_meas : Outport  VectorParamsAs1DForOutWhenUnconnected=off
  wires:
  HP_D_face/1 -> Sum9/2
  HP_D_cell/1 -> Sum9/1
  HP_F_cmd/1 -> Sum1/1
  HpK/1 -> Sum1/2
  Sum1/1 -> HP_F_meas/1
  Sum9/1 -> HpK/1

== system ims_Build5pt1g_tj/M1_HP_loadcells/M1S7 Control ==
  note: HP Relative
      | Displacements
  note: HP Forces
  HP_F_cmd : Inport
  HP_D_cell : Inport  Port=2
  HP_D_face : Inport  Port=3
  HpK : Gain  Gain=m1sys{7}.HPstiff
  Sum1 : Sum  Inputs=-+|
  Sum9 : Sum  Inputs=-+|
  HP_F_meas : Outport  VectorParamsAs1DForOutWhenUnconnected=off
  wires:
  HP_D_face/1 -> Sum9/2
  HP_D_cell/1 -> Sum9/1
  HP_F_cmd/1 -> Sum1/1
  HpK/1 -> Sum1/2
  Sum1/1 -> HP_F_meas/1
  Sum9/1 -> HpK/1

== system ims_Build5pt1g_tj/M2_PZT_Control/PZT Selector ==
  In1 : Inport
  Selector : Selector  InputPortWidth=21  IndexOptions=Index vector (dialog)  Indices=[1:3]  OutputSizes=1
  Selector1 : Selector  InputPortWidth=21  IndexOptions=Index vector (dialog)  Indices=[4:6]  OutputSizes=1
  Selector5 : Selector  InputPortWidth=21  IndexOptions=Index vector (dialog)  Indices=[19:21]  OutputSizes=1
  S1 : Outport  VectorParamsAs1DForOutWhenUnconnected=off
  S2 : Outport  Port=2  VectorParamsAs1DForOutWhenUnconnected=off
  S7 : Outport  Port=3  VectorParamsAs1DForOutWhenUnconnected=off
  wires:
  Selector1/1 -> S2/1
  Selector/1 -> S1/1
  In1/1 -> Selector5/1, Selector1/1, Selector/1
  Selector5/1 -> S7/1

== system ims_Build5pt1g_tj/M2_PZT_Control/PZT selector ==
  In1 : Inport
  Selector : Selector  InputPortWidth=42  IndexOptions=Index vector (dialog)  Indices=[1:6:42]  OutputSizes=1
  Selector1 : Selector  InputPortWidth=42  IndexOptions=Index vector (dialog)  Indices=[2:6:42]  OutputSizes=1
  Selector2 : Selector  InputPortWidth=42  IndexOptions=Index vector (dialog)  Indices=[3:6:42]  OutputSizes=1
  Selector3 : Selector  InputPortWidth=42  IndexOptions=Index vector (dialog)  Indices=[4:6:42]  OutputSizes=1
  Selector4 : Selector  InputPortWidth=42  IndexOptions=Index vector (dialog)  Indices=[5:6:42]  OutputSizes=1
  Selector5 : Selector  InputPortWidth=42  IndexOptions=Index vector (dialog)  Indices=[6:6:42]  OutputSizes=1
  Sum : Sum  Inputs=|+-
  Sum1 : Sum  Inputs=|+-
  Sum2 : Sum  Inputs=|+-
  PZT1 : Outport  VectorParamsAs1DForOutWhenUnconnected=off
  PZT2 : Outport  Port=2  VectorParamsAs1DForOutWhenUnconnected=off
  PZT3 : Outport  Port=3  VectorParamsAs1DForOutWhenUnconnected=off
  wires:
  In1/1 -> Selector1/1, Selector3/1, Selector/1, Selector2/1, Selector5/1, Selector4/1
  Selector/1 -> Sum/1
  Sum/1 -> PZT1/1
  Sum2/1 -> PZT3/1
  Sum1/1 -> PZT2/1
  Selector1/1 -> Sum1/1
  Selector5/1 -> Sum2/2
  Selector2/1 -> Sum2/1
  Selector4/1 -> Sum1/2
  Selector3/1 -> Sum/2

== system ims_Build5pt1g_tj/M2_PZT_Control/PZT selector1 ==
  In1 : Inport
  Selector : Selector  InputPortWidth=42  IndexOptions=Index vector (dialog)  Indices=[1:6:42]  OutputSizes=1
  Selector1 : Selector  InputPortWidth=42  IndexOptions=Index vector (dialog)  Indices=[2:6:42]  OutputSizes=1
  Selector2 : Selector  InputPortWidth=42  IndexOptions=Index vector (dialog)  Indices=[3:6:42]  OutputSizes=1
  Selector3 : Selector  InputPortWidth=42  IndexOptions=Index vector (dialog)  Indices=[4:6:42]  OutputSizes=1
  Selector4 : Selector  InputPortWidth=42  IndexOptions=Index vector (dialog)  Indices=[5:6:42]  OutputSizes=1
  Selector5 : Selector  InputPortWidth=42  IndexOptions=Index vector (dialog)  Indices=[6:6:42]  OutputSizes=1
  Sum : Sum  Inputs=|+-
  Sum1 : Sum  Inputs=|+-
  Sum2 : Sum  Inputs=|+-
  PZT1 : Outport  VectorParamsAs1DForOutWhenUnconnected=off
  PZT2 : Outport  Port=2  VectorParamsAs1DForOutWhenUnconnected=off
  PZT3 : Outport  Port=3  VectorParamsAs1DForOutWhenUnconnected=off
  wires:
  In1/1 -> Selector1/1, Selector3/1, Selector/1, Selector2/1, Selector5/1, Selector4/1
  Selector/1 -> Sum/1
  Selector5/1 -> Sum2/2
  Selector4/1 -> Sum1/2
  Sum1/1 -> PZT2/1
  Sum2/1 -> PZT3/1
  Selector2/1 -> Sum2/1
  Selector3/1 -> Sum/2
  Sum/1 -> PZT1/1
  Selector1/1 -> Sum1/1

== system ims_Build5pt1g_tj/M2_PZT_Control/PZT_Control_FSM1 ==
  PZT_cmd : Inport
  PZT_FB : Inport  Port=2
  Sum : Sum  Inputs=|+-
  multi-rate SS : ims_block_library/multi-rate SS  ss_model=m2pzt{1}.SSdtHfb
  rPZT : Scope  Commented=on
  rel_PZT_D : Gain  Gain=kron(eye(3),[-1,1])  Multiplication=Matrix(K*u)
  spliF_matrix : Gain  Gain=kron(eye(3),[-1;1])  Multiplication=Matrix(K*u)
  m2PZT_u : Outport  VectorParamsAs1DForOutWhenUnconnected=off
  wires:
  Sum/1 -> multi-rate SS/1
  spliF_matrix/1 -> m2PZT_u/1
  PZT_FB/1 -> rel_PZT_D/1
  rel_PZT_D/1 -> Sum/2
  PZT_cmd/1 -> Sum/1
  multi-rate SS/1 -> spliF_matrix/1

== system ims_Build5pt1g_tj/M2_PZT_Control/PZT_Control_FSM2 ==
  PZT_cmd : Inport
  PZT_FB : Inport  Port=2
  Sum : Sum  Inputs=|+-
  multi-rate SS : ims_block_library/multi-rate SS  ss_model=m2pzt{2}.SSdtHfb
  rel_PZT_D : Gain  Gain=kron(eye(3),[-1,1])  Multiplication=Matrix(K*u)
  spliF_matrix : Gain  Gain=kron(eye(3),[-1;1])  Multiplication=Matrix(K*u)
  m2PZT_u : Outport  VectorParamsAs1DForOutWhenUnconnected=off
  wires:
  Sum/1 -> multi-rate SS/1
  spliF_matrix/1 -> m2PZT_u/1
  PZT_FB/1 -> rel_PZT_D/1
  rel_PZT_D/1 -> Sum/2
  PZT_cmd/1 -> Sum/1
  multi-rate SS/1 -> spliF_matrix/1
